simulink model "MPC"  (R2021b)
settings: Solver=VariableStepAuto  StartTime=0.0  StopTime=60  FixedStep=0.02  RelTol=1e-3
model workspace (MAT data in the model file):
  table = [0.138956796593 0.189366832537 0.239777858744 0.290189875214 0.340602881948 0.391016878945 0.441431866206 0.491829747338 0.544679911093 0.601596169389 0.662578522228 0.727626969608 ... (2244 elements, 33x68)]
  table_2 = [0.48 0.587855357616 0.711975093401 0.852359207353 1 1 1 1 1 1 1 1 ... (442 elements, 13x34)]
libraries: Solver_SF x1, simulink x1
settings Model: SimulationMode=accelerator  Creator=JHD  LastModifiedBy=Jing
settings SolverCC: ZeroCrossAlgorithm=Adaptive  AlgebraicLoopSolver=LineSearch
settings DebuggingCC: SFMachineParentedDataDiag=warning

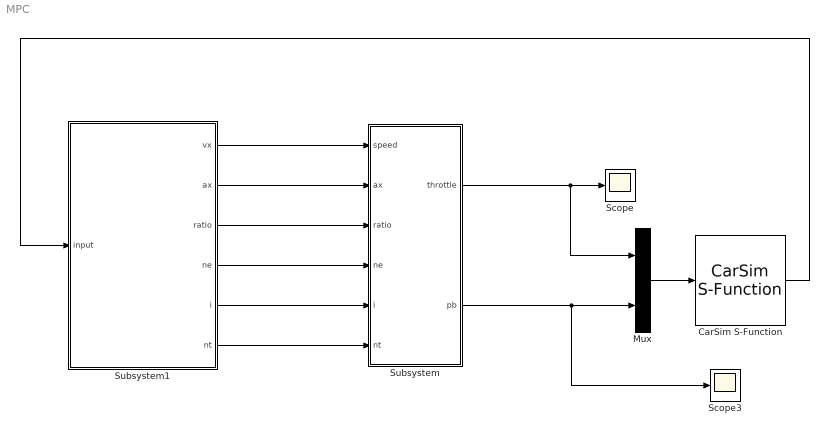
== system MPC ==
  CarSim S-Function : Solver_SF/CarSim S-Function  Priority=1  SIMFILE=simfile.sim
  Mux : Mux  Inputs=2
  Scope : Scope
  Scope3 : Scope
  Subsystem : Subsystem
  Subsystem1 : Subsystem
  wires:
  Mux/1 -> CarSim S-Function/1
  Subsystem/2(pb) -> Scope3/1, Mux/2
  Subsystem/1(throttle) -> Scope/1, Mux/1
  CarSim S-Function/1 -> Subsystem1/1(input)
  Subsystem1/1(vx) -> Subsystem/1(speed)
  Subsystem1/2(ax) -> Subsystem/2(ax)
  Subsystem1/3(ratio) -> Subsystem/3(ratio)
  Subsystem1/4(ne) -> Subsystem/4(ne)
  Subsystem1/5(i) -> Subsystem/5(i)
  Subsystem1/6(nt) -> Subsystem/6(nt)

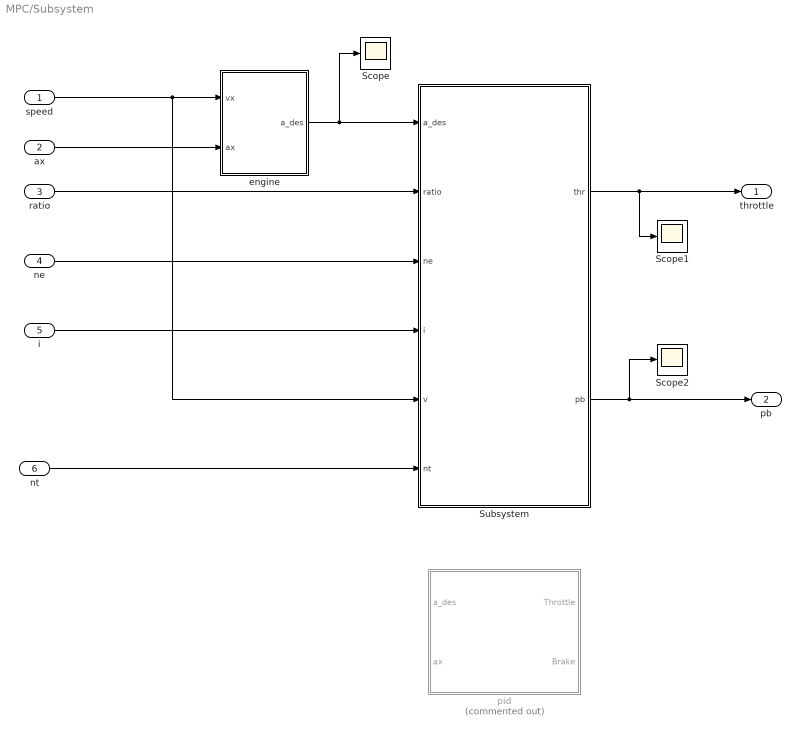
== system MPC/Subsystem ==
  speed : Inport
  ax : Inport  Port=2
  ratio : Inport  Port=3
  ne : Inport  Port=4
  i : Inport  Port=5
  nt : Inport  Port=6
  Scope : Scope
  Scope1 : Scope
  Scope2 : Scope
  Subsystem : Subsystem
  engine : Subsystem
  pid : Subsystem  Commented=on
  throttle : Outport
  pb : Outport  Port=2
  wires:
  ax/1 -> engine/2(ax)
  ratio/1 -> Subsystem/2(ratio)
  ne/1 -> Subsystem/3(ne)
  speed/1 -> engine/1(vx), Subsystem/5(v)
  engine/1(a_des) -> Scope/1, Subsystem/1(a_des)
  Subsystem/1(thr) -> throttle/1, Scope1/1
  Subsystem/2(pb) -> Scope2/1, pb/1
  i/1 -> Subsystem/4(i)
  nt/1 -> Subsystem/6(nt)

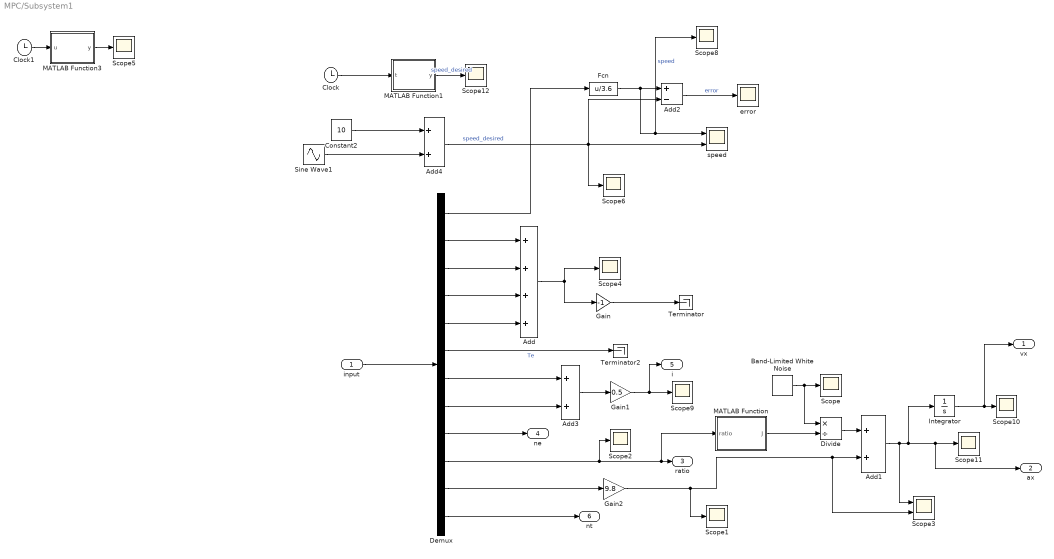
== system MPC/Subsystem1 ==
  input : Inport
  Add : Sum  Inputs=++++
  Add1 : Sum
  Add2 : Sum  Inputs=+-
  Add3 : Sum
  Add4 : Sum
  Band-Limited White Noise : simulink/Sources/Band-Limited White Noise  Cov=[0.5]  Ts=0.1  seed=[23341]
  Clock : Clock
  Clock1 : Clock
  Constant2 : Constant  Value=10
  Demux : Demux  Outputs=12
  Divide : Product  Inputs=*/
  Fcn : Fcn  Expr=u/3.6
  Gain : Gain  Gain=-1
  Gain1 : Gain  Gain=0.5
  Gain2 : Gain  Gain=9.8
  Integrator : Integrator
  MATLAB Function : MATLAB Function  TreatAsAtomicUnit=on
  MATLAB Function1 : MATLAB Function  TreatAsAtomicUnit=on
  MATLAB Function3 : MATLAB Function  TreatAsAtomicUnit=on
  Scope{,1..2,4..6,8..12} (11 alike) : Scope
  Scope3 : Scope  NumInputPorts=2
  Sine Wave1 : Sin  Amplitude=6  Frequency=0.3  Phase=7.5*pi  SampleTime=0
  Terminator : Terminator
  Terminator2 : Terminator
  error : Scope
  speed : Scope  NumInputPorts=2
  vx : Outport
  ax : Outport  Port=2
  ratio : Outport  Port=3
  ne : Outport  Port=4
  i : Outport  Port=5
  nt : Outport  Port=6
  wires:
  Demux/12 -> nt/1
  Demux/11 -> Gain2/1
  Demux/8 -> Add3/2
  Fcn/1 -> Add2/1, Scope8/1, speed/1  "speed"
  Constant2/1 -> Add4/1
  Demux/3 -> Add/2
  Gain2/1 -> Scope3/2, Add1/2, Scope1/1
  Demux/10 -> Scope2/1, MATLAB Function/1(ratio), ratio/1
  Clock/1 -> MATLAB Function1/1(t)
  Demux/6 -> Terminator2/1  "Te"
  Sine Wave1/1 -> Add4/2
  Gain/1 -> Terminator/1
  Demux/9 -> ne/1
  Clock1/1 -> MATLAB Function3/1(u)
  Gain1/1 -> Scope9/1, i/1
  Demux/2 -> Add/1
  Demux/1 -> Fcn/1
  Demux/7 -> Add3/1
  Demux/4 -> Add/3
  Add4/1 -> Scope6/1, Add2/2, speed/2  "speed_desired"
  Demux/5 -> Add/4
  input/1 -> Demux/1
  Add/1 -> Scope4/1, Gain/1
  Add3/1 -> Gain1/1
  MATLAB Function3/1(y) -> Scope5/1
  Add2/1 -> error/1  "error"
  Band-Limited White Noise/1 -> Divide/1, Scope/1
  MATLAB Function/1(J) -> Divide/2
  Divide/1 -> Add1/1
  Add1/1 -> Scope3/1, ax/1, Scope11/1, Integrator/1
  Integrator/1 -> vx/1, Scope10/1
  MATLAB Function1/1(y) -> Scope12/1  "speed_desired"

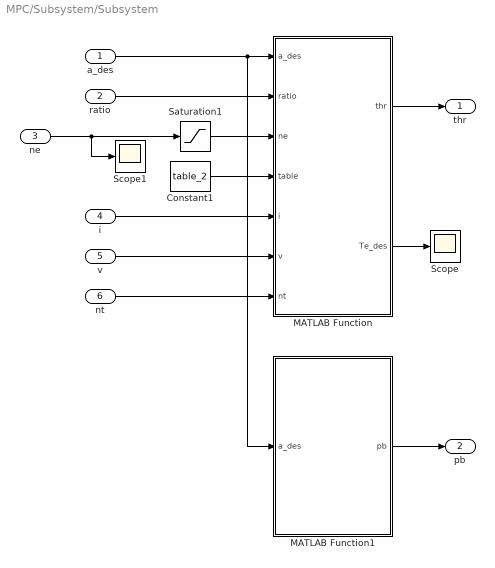
== system MPC/Subsystem/Subsystem ==
  a_des : Inport
  ratio : Inport  Port=2
  ne : Inport  Port=3
  i : Inport  Port=4
  v : Inport  Port=5
  nt : Inport  Port=6
  Constant1 : Constant  Value=table_2
  MATLAB Function : MATLAB Function  TreatAsAtomicUnit=on
  MATLAB Function1 : MATLAB Function  TreatAsAtomicUnit=on
  Saturation1 : Saturate  UpperLimit=6700  LowerLimit=0
  Scope : Scope
  Scope1 : Scope
  thr : Outport
  pb : Outport  Port=2
  wires:
  a_des/1 -> MATLAB Function1/1(a_des), MATLAB Function/1(a_des)
  ratio/1 -> MATLAB Function/2(ratio)
  Saturation1/1 -> MATLAB Function/3(ne)
  Constant1/1 -> MATLAB Function/4(table)
  ne/1 -> Scope1/1, Saturation1/1
  MATLAB Function/1(thr) -> thr/1
  MATLAB Function1/1(pb) -> pb/1
  i/1 -> MATLAB Function/5(i)
  v/1 -> MATLAB Function/6(v)
  MATLAB Function/2(Te_des) -> Scope/1
  nt/1 -> MATLAB Function/7(nt)

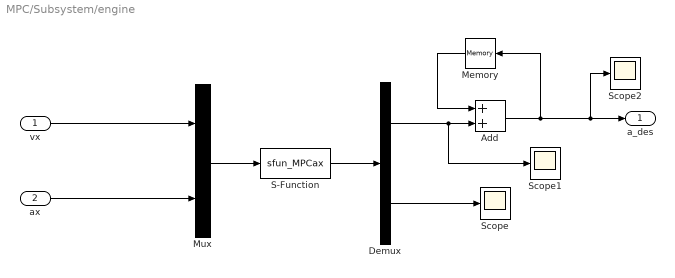
== system MPC/Subsystem/engine ==
  vx : Inport
  ax : Inport  Port=2
  Add : Sum
  Demux : Demux  Outputs=2
  Memory : Memory  InheritSampleTime=on
  Mux : Mux  Inputs=2
  S-Function : S-Function  FunctionName=sfun_MPCax  SFunctionDeploymentMode=off  EnableBusSupport=off
  Scope : Scope
  Scope1 : Scope
  Scope2 : Scope
  a_des : Outport
  wires:
  S-Function/1 -> Demux/1
  Mux/1 -> S-Function/1
  Demux/1 -> Scope1/1, Add/2
  vx/1 -> Mux/1
  ax/1 -> Mux/2
  Demux/2 -> Scope/1
  Add/1 -> Memory/1, Scope2/1, a_des/1
  Memory/1 -> Add/1

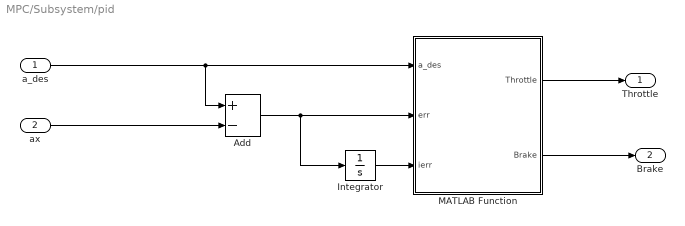
== system MPC/Subsystem/pid ==
  a_des : Inport
  ax : Inport  Port=2
  Add : Sum  Inputs=+-
  Integrator : Integrator
  MATLAB Function : MATLAB Function  TreatAsAtomicUnit=on
  Throttle : Outport
  Brake : Outport  Port=2
  wires:
  Add/1 -> Integrator/1, MATLAB Function/2(err)
  a_des/1 -> MATLAB Function/1(a_des), Add/1
  Integrator/1 -> MATLAB Function/3(ierr)
  MATLAB Function/1(Throttle) -> Throttle/1
  ax/1 -> Add/2
  MATLAB Function/2(Brake) -> Brake/1

== matlab function MPC/Subsystem1/MATLAB Function ==
  data: ratio input; J output
function J = fcn(ratio)

Je=0.16;    % 发动机转动惯量
Jwf=0.9;    % 前后轮转动惯量
Jwr=0.9;
m=1412;
r=0.33;
g=9.8;
f=0.0038;
Cd=0.3;
rou=1.206;
A=2.2;
cx = Cd*rou*A/2;

Rg=1/(4.1*ratio);

J=(Je+Rg*Rg*(Jwf+Jwr+m*r*r))/Rg/r;
end

== matlab function MPC/Subsystem/Subsystem/MATLAB Function ==
  data: a_des input; thr output; ratio input; ne input; table input; i input; v input; Te_des output; nt input
function [thr, Te_des] = fcn(a_des, ratio, ne, table, i, v, nt)

Je=0.16;    % 发动机转动惯量
Jwf=0.9;    % 前后轮转动惯量
Jwr=0.9;
m=1412;
r=0.33;
g=9.8;
f=0.0038;
Cd=0.3;
rou=1.206;
A=2.2;
cx = Cd*rou*A/2;

Rg=1/(4.1*ratio);

J=(Je+Rg*Rg*(Jwf+Jwr+m*r*r))/Rg/r;

% Tc_des = a_des*J + Rg*r*(m*g*f+cx*v^2+m*g*i);
% Tc_des = a_des*J;
Tc_des = a_des*m*r*Rg;

stc = nt/ne;
if stc >= 0.88
    ftr = 1;
else
    ftr = 1.9 - (1.9-1)/0.88*nt/ne;
end
Te_des = Tc_des/ftr;

x = 0:200:6700;
y = 0:20:250;
z = table;

if a_des >= 0
    if Te_des >= 250
        Te_des = 250;
    elseif Te_des <=0
        Te_des = 0;
    else
    end
    thr = interp2(x,y,z,ne,Te_des);
else
    thr = 0;
    Te_des = 0;
end

end

== matlab function MPC/Subsystem/pid/MATLAB Function ==
  data: a_des input; err input; Throttle output; Brake output; ierr input
function [Throttle, Brake] = fcn(a_des, err, ierr)
% 车辆下位控制器将期望加速度转化为油门控制量和制动主缸压力控制量

Brake_Sat = 10;
Throttle_Sat = 1;

kp_thr = 0.3;
ki_thr = 0.05;

kp_brk = -0.4;
ki_brk = -0.1;

if a_des < 0    % Brake control
    Brake = kp_brk * err + ki_brk * ierr;
    if Brake > Brake_Sat
        Brake = Brake_Sat;
    end
    if Brake < 0
        Brake = 0;
    end
    Throttle = 0;
else            % throttle control
    Brake = 0;
    Throttle = kp_thr * err + ki_thr * ierr;
    if Throttle > Throttle_Sat
        Throttle = Throttle_Sat;
    end
    if Throttle < 0
        Throttle = 0;
    end
end

end

== matlab function MPC/Subsystem/Subsystem/MATLAB Function1 ==
  data: a_des input; pb output
function pb = fcn(a_des)


m = 1412;
r = 0.33;

Tb_des = -m*a_des*r;

if a_des >= 0

    pb = 0;
else
    pb = Tb_des/800;
end

end

== matlab function MPC/Subsystem1/MATLAB Function1 ==
  data: t input; y output
function y = fcn(t)

t1 = 8;
t2 = 6;
k1 = 6;
k2 = 4;
T = 60;
k3 = 7.5;
k4 = 5;

if t<t1
    y = 5;
elseif t<pi * k1 + t1
    y = sin((t-pi/2*k1-t1) * 1/k1) * k3 + 5+k3;
elseif t<T-pi*k2-t2
    y= 5 + 2*k3;
elseif t<T-t2
    y = cos(1/k2*(t + pi*k2 -T +t2)) * k4 + 5+2*k3-k4;
else
    y = 5+2*k3-2*k4;
end

end

== matlab function MPC/Subsystem1/MATLAB Function3 ==
  data: u input; y output
function y = fcn(u)

k1 = 10;
T = 60;
k2 = 15;

if u<pi/2 * k1
    y = sin(u * 1/k1) * k2;
else
    if u<T-pi/2*k1
        y=1 * k2;
    else
        y = sin(1/k1*(u - T + pi*k1)) * k2;
    end
end
